simulink model "Automatic_Control1"  (R2021a)
settings: Solver=VariableStepAuto  StartTime=0.0  StopTime=500  RelTol=1e-3
values from neighbouring files (symbols this model uses):
  b = 0.006    [Automatic_Control.m]
  Jm = 0.05    [Automatic_Control.m]
  Ke = 0.05    [Automatic_Control.m]
  Kt = 0.05    [Automatic_Control.m]
  La = 0.01    [Automatic_Control.m]
  Ra = 10    [Automatic_Control.m]
libraries: simulink x1
settings Model: Creator=Rosa  LastModifiedBy=han_jjun_mac
settings SolverCC: AlgebraicLoopSolver=TrustRegion
settings DebuggingCC: SFMachineParentedDataDiag=warning

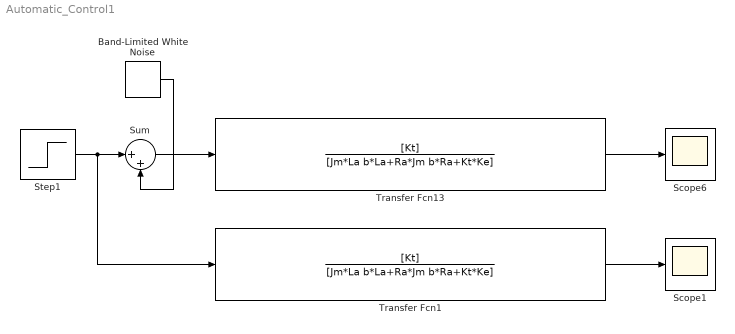
== system Automatic_Control1 ==
  Band-Limited White Noise : simulink/Sources/Band-Limited White Noise  Cov=[1.5]  Ts=0.1  seed=[23341]
  Scope1 : Scope
  Scope6 : Scope
  Step1 : Step  Before=12  After=12  SampleTime=0
  Sum : Sum  Inputs=|++
  Transfer Fcn1 : TransferFcn  Numerator=[Kt]  Denominator=[Jm*La b*La+Ra*Jm b*Ra+Kt*Ke]
  Transfer Fcn13 : TransferFcn  Numerator=[Kt]  Denominator=[Jm*La b*La+Ra*Jm b*Ra+Kt*Ke]
  wires:
  Transfer Fcn13/1 -> Scope6/1
  Sum/1 -> Transfer Fcn13/1
  Band-Limited White Noise/1 -> Sum/2
  Step1/1 -> Transfer Fcn1/1, Sum/1
  Transfer Fcn1/1 -> Scope1/1
